simulink model "Tractive_System_model"  (R2025b)
settings: Solver=ode15s  StartTime=0  StopTime=169.89  MaxStep=1e-3  RelTol=1e-3  AbsTol=1e-6
PreLoadFcn:
  | vehicleData
undefined symbols (not defined in the file): FL, FR, RL, RR, vehicle
libraries: batteryecm_lib x281, fl_lib x86, nesl_utility x54, ee_lib x16, sdl_lib x10, SimscapeFluids_lib x3, BatteryEstimators x2, simulink x1, slpidlib x1, autolibshared x1, eePmsmFieldOrientedControl x1
(part 5 of 26)

== system Tractive_System_model/Cooling system/Subsystem1 ==
  Inverter Power_loss : Scope
      settings: ActiveDisplayYMinimum=494.41730224534911  ActiveDisplayYMaximum=494.45341613974995  DataLoggingVariableName=ScopeData3
  PS Lookup Table (2D) : fl_lib/Physical Signals/Lookup Tables/PS Lookup Table (2D)  x1=[100, 150, 200, 250, 300, 350, 400, 450, 500, 550, 600, 650, 700, 750, 800] V  x2=[100, 150, 200, 250, 300, 350, 400, 450, 500, 550, 600] A  f=|  interp_method=simscape.enum.interpolation.smooth  extrap_method=simscape.enum.extrapolation.nearest
      | [199.5, 318, 436.5, 580.5, 724.5, 899.8, 1075, 1267.5, 1460, 1692.5, 1925;
      | 230.3, 362.3, 494.3, 651.8, 809.3, 998.4, 1187.5, 1393.8, 1600, 1843.8, 2087.5;
      | 261, 406.5, 552, 723, 894, 1097, 1300, 1520, 1740, 1995, 2250;
      | 291.8, 450.8, 609.8, 794.3, 978.8, 1195.6, 1412.5, 1646.3, 1880, 2146.3, 2412.5;
      | 322.5, 495, 667.5, 865.5, 1063.5, 1294.3, 1525, 1772.5, 2020, 2297.5, 2575;
      | 353.3, 539.3, 725.3, 936.8, 1148.3, 1392.9, 1637.5, 1898.8, 2160, 2448.8, 2737.5;
      | 384, 583.5, 783, 1008, 1233, 1491.5, 1750, 2025, 2300, 2600, 2900;
      | 416.3, 629.3, 842.3, 1081.5, 1320.8, 1591.6, 1862.5, 2156.3, 2450, 2768.8, 3087.5;
      | 448.5, 675, 901.5, 1155, 1408.5, 1691.8, 1975, 2287.5, 2600, 2937.5, 3275;
      | 480.8, 720.8, 960.8, 1228.5, 1496.3, 1791.9, 2087.5, 2418.8, 2750, 3106.3, 3462.5;
      | 513, 766.5, 1020, 1302, 1584, 1892, 2200, 2550, 2900, 3275, 3650;
      | 545.3, 812.6, 1080, 1378.5, 1677, 2006, 2335, 2698.8, 3062.5, 3462.5, 3862.5;
      | 577.5, 858.8, 1140, 1455, 1770, 2120, 2470, 2847.5, 3225, 3650, 4075;
      | 609.8, 904.9, 1200, 1531.5, 1863, 2234, 2605, 2996.3, 3387.5, 3837.5, 4287.5;
      | 642, 951, 1260, 1608, 1956, 2348, 2740, 3145, 3550, 4025, 4500] W
  PS-Simulink Converter : nesl_utility/PS-Simulink Converter  PhysicalDomain=network_engine_domain  SubClassName=ps_output  LeftPortType=input  RightPortType=output  PseudoPeriodic=off  Frequencies=[]  VectorFormat=inherit  Unit=W  AffineConversion=off
  PS-Simulink Converter1 : nesl_utility/PS-Simulink Converter  PhysicalDomain=network_engine_domain  SubClassName=ps_output  LeftPortType=input  RightPortType=output  PseudoPeriodic=off  Frequencies=[]  VectorFormat=inherit  Unit=W  AffineConversion=off
  Simulink-PS Converter : nesl_utility/Simulink-PS Converter  PhysicalDomain=network_engine_domain  SubClassName=ps_input  LeftPortType=input  RightPortType=output  PseudoPeriodic=off  Frequencies=[]  NoiseDistribution=none  NoiseParameters=[]  Unit=W  AffineConversion=off  FilteringAndDerivatives=provide  SimscapeFilterOrder=1  InputFilterTimeConstant=0.001  UdotUserProvided=0
  ARMS_IN : PMIOPort  Side=Left
  VDC_IN : PMIOPort  Port=2  Side=Left
  output : PMIOPort  Port=3  Side=Right
  wires:
  PS-Simulink Converter1/1 -> Simulink-PS Converter/1
  PS-Simulink Converter/1 -> Inverter Power_loss/1
  connections:
  Simulink-PS Converter/RConn1 -- output/RConn1
  ARMS_IN/RConn1 -- PS Lookup Table (2D)/LConn2
  VDC_IN/RConn1 -- PS Lookup Table (2D)/LConn1
  PS-Simulink Converter/LConn1 -- PS Lookup Table (2D)/RConn1 -- PS-Simulink Converter1/LConn1

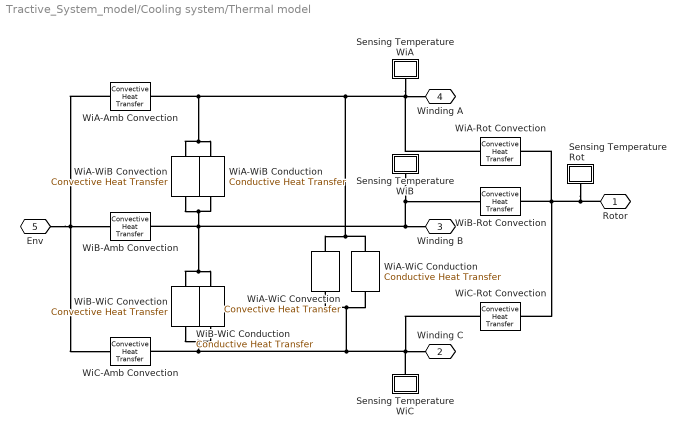
== system Tractive_System_model/Cooling system/Thermal model ==
  Sensing Temperature Rot : Subsystem
      mask Display: disp('TR')
  Sensing Temperature WiA : Subsystem
      mask Display: disp('TA')
  Sensing Temperature WiB : Subsystem
      mask Display: disp('TB')
  Sensing Temperature WiC : Subsystem
      mask Display: disp('TC')
  WiA-Amb Convection : fl_lib/Thermal/Thermal Elements/Convective Heat Transfer  thermal_type=foundation.enum.constant_variable.constant  area=0.1 m^2  heat_tr_coeff=20 W/(m^2 * K)  min_heat_tr_coeff=1e-3 W/(K*m^2)  T_specify=off  T_priority=None  T=0 K  T_nominal_specify=off  T_nominal_value=1  T_nominal_unit=K  Q_specify=off  Q_priority=None  Q=0 J/s  Q_nominal_specify=off  Q_nominal_value=1  Q_nominal_unit=J/s
  WiA-Rot Convection : fl_lib/Thermal/Thermal Elements/Convective Heat Transfer  thermal_type=foundation.enum.constant_variable.constant  area=0.02 m^2  heat_tr_coeff=200 W/(m^2 * K)  min_heat_tr_coeff=1e-3 W/(K*m^2)  T_specify=off  T_priority=None  T=0 K  T_nominal_specify=off  T_nominal_value=1  T_nominal_unit=K  Q_specify=off  Q_priority=None  Q=0 J/s  Q_nominal_specify=off  Q_nominal_value=1  Q_nominal_unit=J/s
  WiA-WiB Conduction : fl_lib/Thermal/Thermal Elements/Conductive Heat Transfer  thermal_type=foundation.enum.ConstantVariableTabulated.Constant  wall_geometry=foundation.enum.ConductionWallGeometry.Planar  area=0.002 m^2  thickness=0.1 m  d_in=0.05 m  d_out=0.1 m  L=1 m  th_cond_min=10 W/(K*m)  th_cond=80 W/(m*K)  th_cond_TLU=[413, 401, 392, 383, 371, 357, 342] W/(K*m)  temp_TLU=[200, 273, 400, 600, 800, 1000, 1200] K  T_specify=off  T_priority=None  T=0 K  T_nominal_specify=off  T_nominal_value=1  T_nominal_unit=K  Q_specify=off  Q_priority=None  Q=0 J/s  Q_nominal_specify=off  Q_nominal_value=1  Q_nominal_unit=J/s
  WiA-WiB Convection : fl_lib/Thermal/Thermal Elements/Convective Heat Transfer  thermal_type=foundation.enum.constant_variable.constant  area=0.004 m^2  heat_tr_coeff=200 W/(m^2 * K)  min_heat_tr_coeff=1e-3 W/(K*m^2)  T_specify=off  T_priority=None  T=0 K  T_nominal_specify=off  T_nominal_value=1  T_nominal_unit=K  Q_specify=off  Q_priority=None  Q=0 J/s  Q_nominal_specify=off  Q_nominal_value=1  Q_nominal_unit=J/s
  WiA-WiC Conduction : fl_lib/Thermal/Thermal Elements/Conductive Heat Transfer  thermal_type=foundation.enum.ConstantVariableTabulated.Constant  wall_geometry=foundation.enum.ConductionWallGeometry.Planar  area=0.002 m^2  thickness=0.1 m  d_in=0.05 m  d_out=0.1 m  L=1 m  th_cond_min=10 W/(K*m)  th_cond=80 W/(m*K)  th_cond_TLU=[413, 401, 392, 383, 371, 357, 342] W/(K*m)  temp_TLU=[200, 273, 400, 600, 800, 1000, 1200] K  T_specify=off  T_priority=None  T=0 K  T_nominal_specify=off  T_nominal_value=1  T_nominal_unit=K  Q_specify=off  Q_priority=None  Q=0 J/s  Q_nominal_specify=off  Q_nominal_value=1  Q_nominal_unit=J/s
  WiA-WiC Convection : fl_lib/Thermal/Thermal Elements/Convective Heat Transfer  thermal_type=foundation.enum.constant_variable.constant  area=0.004 m^2  heat_tr_coeff=200 W/(m^2 * K)  min_heat_tr_coeff=1e-3 W/(K*m^2)  T_specify=off  T_priority=None  T=0 K  T_nominal_specify=off  T_nominal_value=1  T_nominal_unit=K  Q_specify=off  Q_priority=None  Q=0 J/s  Q_nominal_specify=off  Q_nominal_value=1  Q_nominal_unit=J/s
  WiB-Amb Convection : fl_lib/Thermal/Thermal Elements/Convective Heat Transfer  thermal_type=foundation.enum.constant_variable.constant  area=0.1 m^2  heat_tr_coeff=20 W/(m^2 * K)  min_heat_tr_coeff=1e-3 W/(K*m^2)  T_specify=off  T_priority=None  T=0 K  T_nominal_specify=off  T_nominal_value=1  T_nominal_unit=K  Q_specify=off  Q_priority=None  Q=0 J/s  Q_nominal_specify=off  Q_nominal_value=1  Q_nominal_unit=J/s
  WiB-Rot Convection : fl_lib/Thermal/Thermal Elements/Convective Heat Transfer  thermal_type=foundation.enum.constant_variable.constant  area=0.02 m^2  heat_tr_coeff=200 W/(m^2 * K)  min_heat_tr_coeff=1e-3 W/(K*m^2)  T_specify=off  T_priority=None  T=0 K  T_nominal_specify=off  T_nominal_value=1  T_nominal_unit=K  Q_specify=off  Q_priority=None  Q=0 J/s  Q_nominal_specify=off  Q_nominal_value=1  Q_nominal_unit=J/s
  WiB-WiC Conduction : fl_lib/Thermal/Thermal Elements/Conductive Heat Transfer  thermal_type=foundation.enum.ConstantVariableTabulated.Constant  wall_geometry=foundation.enum.ConductionWallGeometry.Planar  area=0.002 m^2  thickness=0.1 m  d_in=0.05 m  d_out=0.1 m  L=1 m  th_cond_min=10 W/(K*m)  th_cond=80 W/(m*K)  th_cond_TLU=[413, 401, 392, 383, 371, 357, 342] W/(K*m)  temp_TLU=[200, 273, 400, 600, 800, 1000, 1200] K  T_specify=off  T_priority=None  T=0 K  T_nominal_specify=off  T_nominal_value=1  T_nominal_unit=K  Q_specify=off  Q_priority=None  Q=0 J/s  Q_nominal_specify=off  Q_nominal_value=1  Q_nominal_unit=J/s
  WiB-WiC Convection : fl_lib/Thermal/Thermal Elements/Convective Heat Transfer  thermal_type=foundation.enum.constant_variable.constant  area=0.004 m^2  heat_tr_coeff=200 W/(m^2 * K)  min_heat_tr_coeff=1e-3 W/(K*m^2)  T_specify=off  T_priority=None  T=0 K  T_nominal_specify=off  T_nominal_value=1  T_nominal_unit=K  Q_specify=off  Q_priority=None  Q=0 J/s  Q_nominal_specify=off  Q_nominal_value=1  Q_nominal_unit=J/s
  WiC-Amb Convection : fl_lib/Thermal/Thermal Elements/Convective Heat Transfer  thermal_type=foundation.enum.constant_variable.constant  area=0.1 m^2  heat_tr_coeff=20 W/(m^2 * K)  min_heat_tr_coeff=1e-3 W/(K*m^2)  T_specify=off  T_priority=None  T=0 K  T_nominal_specify=off  T_nominal_value=1  T_nominal_unit=K  Q_specify=off  Q_priority=None  Q=0 J/s  Q_nominal_specify=off  Q_nominal_value=1  Q_nominal_unit=J/s
  WiC-Rot Convection : fl_lib/Thermal/Thermal Elements/Convective Heat Transfer  thermal_type=foundation.enum.constant_variable.constant  area=0.02 m^2  heat_tr_coeff=200 W/(m^2 * K)  min_heat_tr_coeff=1e-3 W/(K*m^2)  T_specify=off  T_priority=None  T=0 K  T_nominal_specify=off  T_nominal_value=1  T_nominal_unit=K  Q_specify=off  Q_priority=None  Q=0 J/s  Q_nominal_specify=off  Q_nominal_value=1  Q_nominal_unit=J/s
  Rotor : PMIOPort  Side=Left
  Winding C : PMIOPort  Port=2  Side=Right
  Winding B : PMIOPort  Port=3  Side=Right
  Winding A : PMIOPort  Port=4  Side=Right
  Env : PMIOPort  Port=5  Side=Left
  connections:
  WiA-Rot Convection/RConn1 -- WiA-WiC Conduction/RConn1 -- WiA-WiC Convection/RConn1 -- WiA-WiB Convection/LConn1 -- WiA-WiB Conduction/LConn1 -- WiA-Amb Convection/LConn1 -- Sensing Temperature WiA/LConn1 -- Winding A/RConn1
  Rotor/RConn1 -- Sensing Temperature Rot/LConn1 -- WiC-Rot Convection/LConn1 -- WiB-Rot Convection/LConn1 -- WiA-Rot Convection/LConn1
  WiA-WiB Convection/RConn1 -- WiA-WiB Conduction/RConn1 -- Sensing Temperature WiB/LConn1 -- WiB-Rot Convection/RConn1 -- Winding B/RConn1 -- WiB-Amb Convection/LConn1 -- WiB-WiC Conduction/LConn1 -- WiB-WiC Convection/LConn1
  WiC-Rot Convection/RConn1 -- Winding C/RConn1 -- WiB-WiC Conduction/RConn1 -- WiB-WiC Convection/RConn1 -- WiC-Amb Convection/LConn1 -- WiA-WiC Convection/LConn1 -- WiA-WiC Conduction/LConn1 -- Sensing Temperature WiC/LConn1
  WiA-Amb Convection/RConn1 -- Env/RConn1 -- WiC-Amb Convection/RConn1 -- WiB-Amb Convection/RConn1

== system Tractive_System_model/Longitudinal Vehicle Dynamics1/Brakes ==
  Brake FL : sdl_lib/Brakes & Detents/Rotational/Disc Brake  r_mean=brake.padRadius mm  bore=brake.cylinderBore mm  n_pads=1  thermal_port=simscape.enum.thermaleffects.omit  mu_static=brake.sf  mu_coulomb=brake.cf  temperature_TLU=[280, 300, 320] K  mu_static_TLU=[.9, .8, .7]  mu_coulomb_TLU=[.8, .7, .6]  brkwy_vel=brake.frictionVel rad/s  visc_coef=brake.vfc N*m*s/rad  thermal_mass=50 kJ/K  temperature_specify=off  temperature_priority=High  temperature=300 K  temperature_nominal_specify=off  temperature_nominal_value=1  temperature_nominal_unit=K
  Brake FR : sdl_lib/Brakes & Detents/Rotational/Disc Brake  r_mean=brake.padRadius mm  bore=brake.cylinderBore mm  n_pads=1  thermal_port=simscape.enum.thermaleffects.omit  mu_static=brake.sf  mu_coulomb=brake.cf  temperature_TLU=[280, 300, 320] K  mu_static_TLU=[.9, .8, .7]  mu_coulomb_TLU=[.8, .7, .6]  brkwy_vel=brake.frictionVel rad/s  visc_coef=brake.vfc N*m*s/rad  thermal_mass=50 kJ/K  temperature_specify=off  temperature_priority=High  temperature=300 K  temperature_nominal_specify=off  temperature_nominal_value=1  temperature_nominal_unit=K
  Brake RL : sdl_lib/Brakes & Detents/Rotational/Disc Brake  r_mean=brake.padRadius mm  bore=brake.cylinderBore mm  n_pads=1  thermal_port=simscape.enum.thermaleffects.omit  mu_static=brake.sf  mu_coulomb=brake.cf  temperature_TLU=[280, 300, 320] K  mu_static_TLU=[.9, .8, .7]  mu_coulomb_TLU=[.8, .7, .6]  brkwy_vel=brake.frictionVel rad/s  visc_coef=brake.vfc N*m*s/rad  thermal_mass=50 kJ/K  temperature_specify=off  temperature_priority=High  temperature=300 K  temperature_nominal_specify=off  temperature_nominal_value=1  temperature_nominal_unit=K
  Brake RR : sdl_lib/Brakes & Detents/Rotational/Disc Brake  r_mean=brake.padRadius mm  bore=brake.cylinderBore mm  n_pads=1  thermal_port=simscape.enum.thermaleffects.omit  mu_static=brake.sf  mu_coulomb=brake.cf  temperature_TLU=[280, 300, 320] K  mu_static_TLU=[.9, .8, .7]  mu_coulomb_TLU=[.8, .7, .6]  brkwy_vel=brake.frictionVel rad/s  visc_coef=brake.vfc N*m*s/rad  thermal_mass=50 kJ/K  temperature_specify=off  temperature_priority=High  temperature=300 K  temperature_nominal_specify=off  temperature_nominal_value=1  temperature_nominal_unit=K
  Sensing FL : Subsystem
  Sensing FR : Subsystem
  Sensing RL : Subsystem
  Sensing RR : Subsystem
  Simscape Bus : SimscapeBus  HierarchyStrings=RR;RL;FL;FR
  BrakePrF : PMIOPort  Side=Left
  BrakePrR : PMIOPort  Port=2  Side=Left
  Shafts : PMIOPort  Port=3  Side=Right
  Out Bus Element : Outport  PortName=m  Element=FL
  Out Bus Element1 : Outport  PortName=m  Element=FR
  Out Bus Element2 : Outport  PortName=m  Element=RL
  Out Bus Element3 : Outport  PortName=m  Element=RR
  wires:
  Sensing FL/1(m) -> Out Bus Element/1
  Sensing FR/1(m) -> Out Bus Element1/1
  Sensing RL/1(m) -> Out Bus Element2/1
  Sensing RR/1(m) -> Out Bus Element3/1
  connections:
  BrakePrR/RConn1 -- Brake RL/LConn1 -- Brake RR/LConn1
  Brake FR/LConn1 -- Brake FL/LConn1 -- BrakePrF/RConn1
  Sensing FL/LConn1 -- Simscape Bus/LConn3
  Sensing FR/LConn1 -- Simscape Bus/LConn4
  Simscape Bus/LConn2 -- Sensing RL/LConn1
  Sensing RR/LConn1 -- Simscape Bus/LConn1
  Simscape Bus/RConn1 -- Shafts/RConn1
  Sensing FL/RConn1 -- Brake FL/LConn2
  Sensing FR/RConn1 -- Brake FR/LConn2
  Brake RL/LConn2 -- Sensing RL/RConn1
  Sensing RR/RConn1 -- Brake RR/LConn2

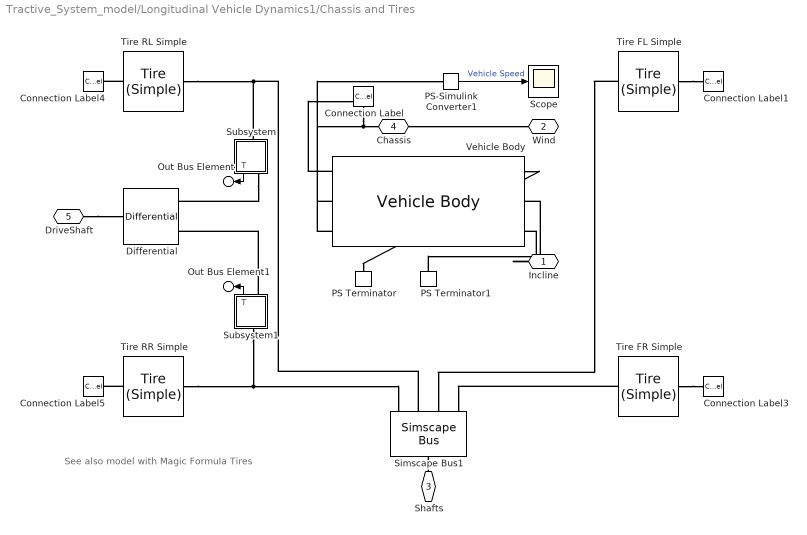
== system Tractive_System_model/Longitudinal Vehicle Dynamics1/Chassis and Tires ==
  note: See also model with Magic Formula Tires
  Connection Label{,1,3..5} (5 alike) : ConnectionLabel  Label=VehicleHub
  Differential : sdl_lib/Gears/Differential  driveshaft_location=sdl.enum.differential_orientation.right  cd_ratio=4.28  friction_model=sdl.enum.gear_friction.none  efficiency=[.85, .92]  temperature_TLU=[280, 300, 320] K  efficiency_ss_TLU=[.95, .9, .85]  efficiency_cd_TLU=[.95, .9, .85]  pwr_thr=[.001, .001] W  mu_visc=[0, 0] N*m*s/rad  model_inertia=simscape.enum.onoff.off  sun_inertia=1e-10 kg*m^2  sun_radius=0.01 m  carrier_inertia=0.001 kg*m^2  planet_inertia=0.001 kg*m^2  planet_mass=1e-10 kg  thermal_mass=50 J/K  T_init=300 K
  PS Terminator : fl_lib/Physical Signals/Sinks/PS Terminator
  PS Terminator1 : fl_lib/Physical Signals/Sinks/PS Terminator
  PS-Simulink Converter1 : nesl_utility/PS-Simulink Converter  PhysicalDomain=network_engine_domain  SubClassName=ps_output  LeftPortType=input  RightPortType=output  PseudoPeriodic=off  Frequencies=[]  VectorFormat=1-D array  Unit=1  AffineConversion=off
  Scope : Scope
      settings: ActiveDisplayYMinimum=-3.15304  ActiveDisplayYMaximum=29.55672  DataLoggingSaveFormat=Array
  Simscape Bus1 : SimscapeBus  HierarchyStrings=RR;RL;FL;FR
  Subsystem : Subsystem
  Subsystem1 : Subsystem
  Tire FL Simple : sdl_lib/Tires & Vehicles/Tire (Simple)  r_tire=vehicle.tireRollingRadius_cm cm  model_compliance=sdl.enum.compliance.off  stiffness=1e6 N/m  damping=1000 N*s/m  model_inertia=sdl.enum.model_inertia.off  tire_inertia=0.01 kg*m^2  initial_velocity=1 rad/s
      settings: InternalSimscapePortConfiguration="{\"Bottom\":[],\"Left\":[{\"id\":\"A\",\"label\":\"A\",\"type\":\"foundation.mechanical.rotational.rotational\"}],\"Right\":[{\"id\":\"H\",\"label\":\"H\",\"type\":\"foundation.mechanical.translational.translational\"}],\"Top\":[]}"
  Tire FR Simple : sdl_lib/Tires & Vehicles/Tire (Simple)  r_tire=vehicle.tireRollingRadius_cm cm  model_compliance=sdl.enum.compliance.off  stiffness=1e6 N/m  damping=1000 N*s/m  model_inertia=sdl.enum.model_inertia.off  tire_inertia=0.01 kg*m^2  initial_velocity=1 rad/s
      settings: InternalSimscapePortConfiguration="{\"Bottom\":[],\"Left\":[{\"id\":\"A\",\"label\":\"A\",\"type\":\"foundation.mechanical.rotational.rotational\"}],\"Right\":[{\"id\":\"H\",\"label\":\"H\",\"type\":\"foundation.mechanical.translational.translational\"}],\"Top\":[]}"
  Tire RL Simple : sdl_lib/Tires & Vehicles/Tire (Simple)  r_tire=vehicle.tireRollingRadius_cm cm  model_compliance=sdl.enum.compliance.off  stiffness=1e6 N/m  damping=1000 N*s/m  model_inertia=sdl.enum.model_inertia.off  tire_inertia=0.01 kg*m^2  initial_velocity=1 rad/s
      settings: InternalSimscapePortConfiguration="{\"Bottom\":[],\"Left\":[{\"id\":\"A\",\"label\":\"A\",\"type\":\"foundation.mechanical.rotational.rotational\"}],\"Right\":[{\"id\":\"H\",\"label\":\"H\",\"type\":\"foundation.mechanical.translational.translational\"}],\"Top\":[]}"
  Tire RR Simple : sdl_lib/Tires & Vehicles/Tire (Simple)  r_tire=vehicle.tireRollingRadius_cm cm  model_compliance=sdl.enum.compliance.off  stiffness=1e6 N/m  damping=1000 N*s/m  model_inertia=sdl.enum.model_inertia.off  tire_inertia=0.01 kg*m^2  initial_velocity=1 rad/s
      settings: InternalSimscapePortConfiguration="{\"Bottom\":[],\"Left\":[{\"id\":\"A\",\"label\":\"A\",\"type\":\"foundation.mechanical.rotational.rotational\"}],\"Right\":[{\"id\":\"H\",\"label\":\"H\",\"type\":\"foundation.mechanical.translational.translational\"}],\"Top\":[]}"
  Vehicle Body : sdl_lib/Tires & Vehicles/Vehicle Body  mass=vehicle.riderMass + vehicle.vehicleMass kg  n_w=2  x_f=vehicle.frontAxleDis mm  x_r=vehicle.rearAxleDis mm  y_c=vehicle.cgHeight mm  mass_var=simscape.enum.onoff.off  g=9.81 m/s^2  liftoff_warning=simscape.enum.onoff.off  area=1 m^2  Cd_var=false  Cd=0  rho=1.18 kg/m^3  model_pitch=simscape.enum.onoff.off  inertia=4000 kg*m^2  suspension_model=sdl.enum.linearTLU.linear  k_f=1e4 N/m  b_f=1e4 N*s/m  k_r=1e4 N/m  b_r=1e4 N*s/m  k_f_TLU=[-2000, -1000, 0, 1000, 2000] N  x_f_TLU=[-.4, -.2, 0, .2, .4] m  b_f_TLU=[-200, -100, 0, 100, 200] N  v_f_TLU=[-4, -2, 0, 2, 4] m/s  k_r_TLU=[-2000, -1000, 0, 1000, 2000] N  x_r_TLU=[-.4, -.2, 0, .2, .4] m  b_r_TLU=[-200, -100, 0, 100, 200] N  v_r_TLU=[-4, -2, 0, 2, 4] m/s  interp_method=simscape.enum.interpolation.linear  extrap_method=simscape.enum.extrapolation.linear  model_hardstop=simscape.enum.onoff.off  upper_bound_f=.25 m  lower_bound_f=-.25 m  stop_k_f=1e6 N/m  stop_b_f=150 N*s/m  upper_bound_r=.25 m  lower_bound_r=-.25 m  stop_k_r=1e6 N/m  stop_b_r=150 N*s/m  initial_pitch=0 rad  initial_pitch_rate=0 rad/s  v_specify=off  v_priority=High  v=12.95 m/s  v_nominal_specify=off  v_nominal_value=1  v_nominal_unit=m/s
      settings: InternalSimscapePortConfiguration="{\"Bottom\":[{\"id\":\"NR\",\"label\":\"NR\",\"type\":\"output\"},{\"id\":\"NF\",\"label\":\"NF\",\"type\":\"output\"},{\"id\":\"beta\",\"label\":\"beta\",\"type\":\"input\"}],\"Left\":[{\"id\":\"H\",\"label\":\"H\",\"type\":\"foundation.mechanical.translational.translational\"}],\"Right\":[],\"Top\":[{\"id\":\"V\",\"label\":\"V\",\"type\":\"output\"},{\"id\":\"wind\",\"label\":\"W\",\"type\":\"input\"}]}"
  Incline : PMIOPort  Side=Right
  Wind : PMIOPort  Port=2  Side=Right
  Shafts : PMIOPort  Port=3  Side=Left
  Chassis : PMIOPort  Port=4  Side=Right
  DriveShaft : PMIOPort  Port=5  Side=Left
  Out Bus Element : Outport  PortName=m  Element=tRL
  Out Bus Element1 : Outport  PortName=m  Element=tRR
  wires:
  PS-Simulink Converter1/1 -> Scope/1  "Vehicle Speed"
  Subsystem/1(T) -> Out Bus Element/1
  Subsystem1/1(T) -> Out Bus Element1/1
  connections:
  Tire RR Simple/RConn1 -- Connection Label5/LConn1
  Tire FL Simple/RConn1 -- Connection Label1/LConn1
  Tire RL Simple/RConn1 -- Connection Label4/LConn1
  Vehicle Body/LConn2 -- PS-Simulink Converter1/LConn1
  Tire FR Simple/RConn1 -- Connection Label3/LConn1
  Tire FR Simple/LConn1 -- Simscape Bus1/LConn4
  DriveShaft/RConn1 -- Differential/LConn1
  Connection Label/LConn1 -- Vehicle Body/LConn1 -- Chassis/RConn1
  Subsystem1/LConn1 -- Tire RR Simple/LConn1 -- Simscape Bus1/LConn1
  Tire FL Simple/LConn1 -- Simscape Bus1/LConn3
  Simscape Bus1/LConn2 -- Tire RL Simple/LConn1 -- Subsystem/LConn1
  Shafts/RConn1 -- Simscape Bus1/RConn1
  Incline/RConn1 -- Vehicle Body/RConn3
  Vehicle Body/LConn3 -- Wind/RConn1
  Subsystem1/RConn1 -- Differential/RConn1
  Subsystem/RConn1 -- Differential/RConn2
  Vehicle Body/RConn1 -- PS Terminator/LConn1
  PS Terminator1/LConn1 -- Vehicle Body/RConn2

== system Tractive_System_model/Longitudinal Vehicle Dynamics1/Env ==
  m : Inport
  Road Grade (rad) : Constant  Value=0
  Signal Specification : SignalSpecification  Unit=rad
  Terminator : Terminator
  Wind (m/s) : Constant  Value=0
  Bus Element Out2 : Outport  PortName=Env  Element=RoadGrade
      settings: AttributesFormatString=%<Unit>
  Bus Element Out4 : Outport  PortName=Env  Element=Wind
      settings: AttributesFormatString=%<Unit>
  wires:
  Wind (m/s)/1 -> Bus Element Out4/1
  m/1 -> Terminator/1
  Road Grade (rad)/1 -> Signal Specification/1
  Signal Specification/1 -> Bus Element Out2/1

== system Tractive_System_model/Longitudinal Vehicle Dynamics1/Sensor Subsystem ==
  AutoTerm : Terminator
  AutoTerm1 : Terminator
  Ideal Translational Motion Sensor : fl_lib/Mechanical/Mechanical Sensors/Ideal Translational Motion Sensor  reference=foundation.enum.MeasurementReference.difference  acceleration_port=false  velocity_port=true  position_port=true  offset=0 m
  Mechanical Translational Reference : fl_lib/Mechanical/Translational Elements/Mechanical Translational Reference
  PS-Simulink Converter1 : nesl_utility/PS-Simulink Converter  PhysicalDomain=network_engine_domain  SubClassName=ps_output  LeftPortType=input  RightPortType=output  PseudoPeriodic=off  Frequencies=[]  VectorFormat=1-D array  Unit=km/hr  AffineConversion=off
  PS-Simulink Converter2 : nesl_utility/PS-Simulink Converter  PhysicalDomain=network_engine_domain  SubClassName=ps_output  LeftPortType=input  RightPortType=output  PseudoPeriodic=off  Frequencies=[]  VectorFormat=1-D array  Unit=1  AffineConversion=off
  PS-Simulink Converter3 : nesl_utility/PS-Simulink Converter  PhysicalDomain=network_engine_domain  SubClassName=ps_output  LeftPortType=input  RightPortType=output  PseudoPeriodic=off  Frequencies=[]  VectorFormat=1-D array  Unit=mph  AffineConversion=off
  PS-Simulink Converter4 : nesl_utility/PS-Simulink Converter  PhysicalDomain=network_engine_domain  SubClassName=ps_output  LeftPortType=input  RightPortType=output  PseudoPeriodic=off  Frequencies=[]  VectorFormat=1-D array  Unit=m/s  AffineConversion=off
  Vehicle : PMIOPort  Side=Left
  kph : Outport  VectorParamsAs1DForOutWhenUnconnected=off
  m/s : Outport  Port=2  VectorParamsAs1DForOutWhenUnconnected=off
  wires:
  PS-Simulink Converter1/1 -> kph/1
  PS-Simulink Converter2/1 -> AutoTerm/1
  PS-Simulink Converter3/1 -> AutoTerm1/1
  PS-Simulink Converter4/1 -> m/s/1
  connections:
  Mechanical Translational Reference/LConn1 -- Ideal Translational Motion Sensor/RConn1
  PS-Simulink Converter2/LConn1 -- Ideal Translational Motion Sensor/RConn3
  Ideal Translational Motion Sensor/LConn1 -- Vehicle/RConn1
  PS-Simulink Converter3/LConn1 -- PS-Simulink Converter4/LConn1 -- Ideal Translational Motion Sensor/RConn2 -- PS-Simulink Converter1/LConn1

== system Tractive_System_model/Referenced battery pack /Accumalator ==
  Module  four : Subsystem
  Module Five1 : Subsystem
  Module One1 : Subsystem
  Module Three1 : Subsystem
  "Module Two " : Subsystem
  - : PMIOPort  Side=Left
  + : PMIOPort  Port=2  Side=Left
  connections:
  Module One1/LConn1 -- +/RConn1
  Module Five1/LConn2 -- -/RConn1
  Module  four/LConn2 -- Module Five1/LConn1
  Module One1/LConn2 -- "Module Two "/LConn1
  Module Three1/LConn2 -- Module  four/LConn1
  "Module Two "/LConn2 -- Module Three1/LConn1

== system Tractive_System_model/Referenced battery pack /SOC1 ==
  Constant2 : Constant
  Current Sensor : fl_lib/Electrical/Electrical Sensors/Current Sensor
  PS-Simulink Converter1 : nesl_utility/PS-Simulink Converter  PhysicalDomain=network_engine_domain  SubClassName=ps_output  LeftPortType=input  RightPortType=output  PseudoPeriodic=off  Frequencies=[]  VectorFormat=inherit  Unit=inherit  AffineConversion=off
  SOC : Scope
      settings: ActiveDisplayYMinimum=-1  ActiveDisplayYMaximum=1  DataLoggingVariableName=ScopeData12
  SOC Estimator (Coulomb Counting) : BatteryEstimators/SOC Estimator (Coulomb Counting)  CurrentInputPartition=on  AH=27  Ts=1  DataType=Inherit: auto
      settings: LibrarySourceBlock=|
      | batt_sl_lib/Estimators/SOC Estimator
      | (Coulomb Counting)
  Conn1 : PMIOPort  Side=Left
  Conn2 : PMIOPort  Port=2  Side=Right
  SOC batt : Outport
  wires:
  Constant2/1 -> SOC Estimator (Coulomb Counting)/2
  SOC Estimator (Coulomb Counting)/1 -> SOC/1, SOC batt/1  "Coulomb counting"
  PS-Simulink Converter1/1 -> SOC Estimator (Coulomb Counting)/1
  connections:
  Current Sensor/LConn1 -- Conn1/RConn1
  Current Sensor/RConn2 -- Conn2/RConn1
  PS-Simulink Converter1/LConn1 -- Current Sensor/RConn1

== system Tractive_System_model/Throttle controller/ Torque Reference ==
  Throtte Positon : Inport  Unit=km/hr
  Constant : Constant  Value=240
  Divide : Product  Inputs=*/
  From Workspace : FromWorkspace  Commented=on  VariableName=Current_Matrix
  Gain : Gain  Gain=0.57735026919
  Gain1 : Gain  Gain=0.83
  Product : Product
  Torque ref : Scope
      settings: ActiveDisplayYMinimum=-13.959117073448896  ActiveDisplayYMaximum=125.63205366104009  DataLoggingVariableName=ScopeData11
  percentage : Constant  Value=100
  Motortrqref : Outport  Unit=rpm  VectorParamsAs1DForOutWhenUnconnected=off
  wires:
  Throtte Positon/1 -> Divide/1
  percentage/1 -> Divide/2
  Divide/1 -> Product/2
  Constant/1 -> Product/1
  Product/1 -> Gain/1
  Gain/1 -> Gain1/1
  Gain1/1 -> Torque ref/1, Motortrqref/1

== system Tractive_System_model/Throttle controller/Control ==
  note: Is Pressure an output?
  Torque Ref : Inport
  motorspd : Inport  Port=2
  bus voltage : Inport  Port=3
  SOC : Inport  Port=4
  20Hz Lowpass Filter : TransferFcn  Denominator=[1/(2*pi*20) 1]
  Cmd Torque : Scope
      settings: ActiveDisplayYMinimum=-13.959117072781753  ActiveDisplayYMaximum=125.6320536550358
  Motor Torque : Subsystem
  MotCmdTrq : Outport
  wires:
  Motor Torque/1(motTrq) -> 20Hz Lowpass Filter/1  "MotCmdTrq"
  SOC/1 -> Motor Torque/2(SOC)
  bus voltage/1 -> Motor Torque/3(bus voltage)
  motorspd/1 -> Motor Torque/4(motorspd)
  Torque Ref/1 -> Motor Torque/1(trqReq)
  20Hz Lowpass Filter/1 -> Cmd Torque/1, MotCmdTrq/1  "Motor Speed"

== system Tractive_System_model/Controller/Control/Brake Force ==
  note: Convert requested braking torque to brake pressure
  trqReq : Inport
  Only Negative Trq : Saturate  UpperLimit=0  LowerLimit=-inf  ZeroCross=off
  trq2pressure : Gain  Gain=-3.3e6
  brkPr : Outport
  wires:
  Only Negative Trq/1 -> trq2pressure/1
  trq2pressure/1 -> brkPr/1
  trqReq/1 -> Only Negative Trq/1  "trqReq"

== system Tractive_System_model/Controller/Control/Motor Torque ==
  note: Check for Gain for regen
  note: Full torque for acceleration,
      | limited torque for deceleration (regenerative torque)
  trqReq : Inport
  1-D Lookup Table : Lookup_n-D  Commented=on  NumberOfTableDimensions=1  BreakpointsForDimension1=[0,8,15,999]  Table=[0,0,1,1]  InternalRulePriority=Speed  RndMeth=Simplest
  1-D Lookup Table1 : Lookup_n-D  Commented=on  NumberOfTableDimensions=1  BreakpointsForDimension1=[0,540,560,999]  Table=[1,1,0,0]  InternalRulePriority=Speed  RndMeth=Simplest
  1-D Lookup Table2 : Lookup_n-D  Commented=on  NumberOfTableDimensions=1  BreakpointsForDimension1=[0,0.8,0.95,1]  Table=[1,1,0,0]  InternalRulePriority=Speed  RndMeth=Simplest
  Compare To Zero : simulink/Logic and Bit Operations/Compare To Zero  relop=>  OutDataTypeStr=boolean  ZeroCross=off
  Gain accel torque : Constant
  Gain decel torque : Constant  Value=0.3
  Product : Product
  Saturation Motor Torque Limits : Saturate  UpperLimit=150  LowerLimit=-150  ZeroCross=off
  Switch : Switch  Criteria=u2 > Threshold  SaturateOnIntegerOverflow=off  InputSameDT=off
  motTrq : Outport
  wires:
  Switch/1 -> Product/1
  Gain accel torque/1 -> Switch/1
  Compare To Zero/1 -> Switch/2
  trqReq/1 -> Product/2, Compare To Zero/1
  Product/1 -> Saturation Motor Torque Limits/1
  Saturation Motor Torque Limits/1 -> motTrq/1
  Gain decel torque/1 -> Switch/3
  1-D Lookup Table/1 -> ?
  1-D Lookup Table1/1 -> ?
  1-D Lookup Table2/1 -> ?

== system Tractive_System_model/Cooling system/Cooling system /Sensing Temperature Inverter ==
  PS-Simulink Converter : nesl_utility/PS-Simulink Converter  PhysicalDomain=network_engine_domain  SubClassName=ps_output  LeftPortType=input  RightPortType=output  PseudoPeriodic=off  Frequencies=[]  VectorFormat=1-D array  Unit=degC  AffineConversion=on
  Temperature Sensor : fl_lib/Thermal/Thermal Sensors/Temperature Sensor  temperature_measure=foundation.enum.MeasurementReference.difference
  ThRef : fl_lib/Thermal/Thermal Elements/Thermal Reference
  H : PMIOPort  Side=Left
  Cooling Inverter : Outport
  wires:
  PS-Simulink Converter/1 -> Cooling Inverter/1
  connections:
  ThRef/LConn1 -- Temperature Sensor/RConn1
  H/RConn1 -- Temperature Sensor/LConn1
  Temperature Sensor/RConn2 -- PS-Simulink Converter/LConn1

== system Tractive_System_model/Cooling system/Cooling system /Subsystem ==
  "Motor Temp " : Scope
      settings: ActiveDisplayYMinimum=24.999993193295392  ActiveDisplayYMaximum=25.000005404995338  DataLoggingVariableName=ScopeData2
  PS-Simulink Converter : nesl_utility/PS-Simulink Converter  PhysicalDomain=network_engine_domain  SubClassName=ps_output  LeftPortType=input  RightPortType=output  PseudoPeriodic=off  Frequencies=[]  VectorFormat=inherit  Unit=degC  AffineConversion=on
  Temperature Sensor : fl_lib/Thermal/Thermal Sensors/Temperature Sensor  temperature_measure=foundation.enum.MeasurementReference.difference
  Thermal Reference : fl_lib/Thermal/Thermal Elements/Thermal Reference
  Conn1 : PMIOPort  Side=Left
  wires:
  PS-Simulink Converter/1 -> "Motor Temp "/1  "Motor Temperature"
  connections:
  Temperature Sensor/LConn1 -- Conn1/RConn1
  Thermal Reference/LConn1 -- Temperature Sensor/RConn1
  PS-Simulink Converter/LConn1 -- Temperature Sensor/RConn2

== system Tractive_System_model/Cooling system/Thermal model/Sensing Temperature Rot ==
  PS-Simulink Converter : nesl_utility/PS-Simulink Converter  PhysicalDomain=network_engine_domain  SubClassName=ps_output  LeftPortType=input  RightPortType=output  PseudoPeriodic=off  Frequencies=[]  VectorFormat=1-D array  Unit=degC  AffineConversion=on
  Temperature Sensor : fl_lib/Thermal/Thermal Sensors/Temperature Sensor  temperature_measure=foundation.enum.MeasurementReference.difference
  ThRef : fl_lib/Thermal/Thermal Elements/Thermal Reference
  H : PMIOPort  Side=Left
  tag scope: TR=global
  wires:
  PS-Simulink Converter/1 -> [TR]
  connections:
  Temperature Sensor/RConn2 -- PS-Simulink Converter/LConn1
  ThRef/LConn1 -- Temperature Sensor/RConn1
  H/RConn1 -- Temperature Sensor/LConn1

== system Tractive_System_model/Cooling system/Thermal model/Sensing Temperature WiA ==
  PS-Simulink Converter : nesl_utility/PS-Simulink Converter  PhysicalDomain=network_engine_domain  SubClassName=ps_output  LeftPortType=input  RightPortType=output  PseudoPeriodic=off  Frequencies=[]  VectorFormat=1-D array  Unit=degC  AffineConversion=on
  Temperature Sensor : fl_lib/Thermal/Thermal Sensors/Temperature Sensor  temperature_measure=foundation.enum.MeasurementReference.difference
  ThRef : fl_lib/Thermal/Thermal Elements/Thermal Reference
  H : PMIOPort  Side=Left
  tag scope: TA=global
  wires:
  PS-Simulink Converter/1 -> [TA]
  connections:
  H/RConn1 -- Temperature Sensor/LConn1
  ThRef/LConn1 -- Temperature Sensor/RConn1
  Temperature Sensor/RConn2 -- PS-Simulink Converter/LConn1

== system Tractive_System_model/Cooling system/Thermal model/Sensing Temperature WiB ==
  PS-Simulink Converter : nesl_utility/PS-Simulink Converter  PhysicalDomain=network_engine_domain  SubClassName=ps_output  LeftPortType=input  RightPortType=output  PseudoPeriodic=off  Frequencies=[]  VectorFormat=1-D array  Unit=degC  AffineConversion=on
  Temperature Sensor : fl_lib/Thermal/Thermal Sensors/Temperature Sensor  temperature_measure=foundation.enum.MeasurementReference.difference
  ThRef : fl_lib/Thermal/Thermal Elements/Thermal Reference
  H : PMIOPort  Side=Left
  tag scope: TB=global
  wires:
  PS-Simulink Converter/1 -> [TB]
  connections:
  ThRef/LConn1 -- Temperature Sensor/RConn1
  H/RConn1 -- Temperature Sensor/LConn1
  Temperature Sensor/RConn2 -- PS-Simulink Converter/LConn1

== system Tractive_System_model/Cooling system/Thermal model/Sensing Temperature WiC ==
  PS-Simulink Converter : nesl_utility/PS-Simulink Converter  PhysicalDomain=network_engine_domain  SubClassName=ps_output  LeftPortType=input  RightPortType=output  PseudoPeriodic=off  Frequencies=[]  VectorFormat=1-D array  Unit=degC  AffineConversion=on
  Temperature Sensor : fl_lib/Thermal/Thermal Sensors/Temperature Sensor  temperature_measure=foundation.enum.MeasurementReference.difference
  ThRef : fl_lib/Thermal/Thermal Elements/Thermal Reference
  H : PMIOPort  Side=Left
  tag scope: TC=global
  wires:
  PS-Simulink Converter/1 -> [TC]
  connections:
  H/RConn1 -- Temperature Sensor/LConn1
  ThRef/LConn1 -- Temperature Sensor/RConn1
  Temperature Sensor/RConn2 -- PS-Simulink Converter/LConn1

== system Tractive_System_model/Longitudinal Vehicle Dynamics1/Brakes/Sensing FL ==
  Mechanical Rotational Reference : fl_lib/Mechanical/Rotational Elements/Mechanical Rotational Reference
  Motion Sensor : fl_lib/Mechanical/Mechanical Sensors/Ideal Rotational Motion Sensor  reference=foundation.enum.MeasurementReference.difference  acceleration_port=false  velocity_port=true  position_port=true  wrap_angle=simscape.enum.onoff.off  offset=0 rad
  PS Terminator : fl_lib/Physical Signals/Sinks/PS Terminator
  PS-Simulink Converter : nesl_utility/PS-Simulink Converter  PhysicalDomain=network_engine_domain  SubClassName=ps_output  LeftPortType=input  RightPortType=output  PseudoPeriodic=off  Frequencies=[]  VectorFormat=inherit  Unit=inherit  AffineConversion=off
  PS-Simulink Converter1 : nesl_utility/PS-Simulink Converter  PhysicalDomain=network_engine_domain  SubClassName=ps_output  LeftPortType=input  RightPortType=output  PseudoPeriodic=off  Frequencies=[]  VectorFormat=inherit  Unit=inherit  AffineConversion=off
  Torque Sensor : fl_lib/Mechanical/Mechanical Sensors/Ideal Torque Sensor
  C : PMIOPort  Side=Left
  R : PMIOPort  Port=2  Side=Right
  Out Bus Element : Outport  PortName=m  Element=brkTrqFL
  Out Bus Element1 : Outport  PortName=m  Element=wFL
  wires:
  PS-Simulink Converter1/1 -> Out Bus Element1/1  "w"
  PS-Simulink Converter/1 -> Out Bus Element/1  "trq"
  connections:
  Motion Sensor/RConn3 -- PS Terminator/LConn1
  PS-Simulink Converter1/LConn1 -- Motion Sensor/RConn2
  Motion Sensor/RConn1 -- Mechanical Rotational Reference/LConn1
  Torque Sensor/RConn1 -- C/RConn1
  Motion Sensor/LConn1 -- Torque Sensor/LConn1 -- R/RConn1
  PS-Simulink Converter/LConn1 -- Torque Sensor/RConn2

== system Tractive_System_model/Longitudinal Vehicle Dynamics1/Brakes/Sensing FR ==
  Mechanical Rotational Reference : fl_lib/Mechanical/Rotational Elements/Mechanical Rotational Reference
  Motion Sensor : fl_lib/Mechanical/Mechanical Sensors/Ideal Rotational Motion Sensor  reference=foundation.enum.MeasurementReference.difference  acceleration_port=false  velocity_port=true  position_port=true  wrap_angle=simscape.enum.onoff.off  offset=0 rad
  PS Terminator : fl_lib/Physical Signals/Sinks/PS Terminator
  PS-Simulink Converter : nesl_utility/PS-Simulink Converter  PhysicalDomain=network_engine_domain  SubClassName=ps_output  LeftPortType=input  RightPortType=output  PseudoPeriodic=off  Frequencies=[]  VectorFormat=inherit  Unit=inherit  AffineConversion=off
  PS-Simulink Converter1 : nesl_utility/PS-Simulink Converter  PhysicalDomain=network_engine_domain  SubClassName=ps_output  LeftPortType=input  RightPortType=output  PseudoPeriodic=off  Frequencies=[]  VectorFormat=inherit  Unit=inherit  AffineConversion=off
  Torque Sensor : fl_lib/Mechanical/Mechanical Sensors/Ideal Torque Sensor
  C : PMIOPort  Side=Left
  R : PMIOPort  Port=2  Side=Right
  Out Bus Element : Outport  PortName=m  Element=brkTrqFR
  Out Bus Element1 : Outport  PortName=m  Element=wFR
  wires:
  PS-Simulink Converter/1 -> Out Bus Element/1  "trq"
  PS-Simulink Converter1/1 -> Out Bus Element1/1  "w"
  connections:
  PS-Simulink Converter/LConn1 -- Torque Sensor/RConn2
  R/RConn1 -- Torque Sensor/LConn1 -- Motion Sensor/LConn1
  Torque Sensor/RConn1 -- C/RConn1
  Motion Sensor/RConn1 -- Mechanical Rotational Reference/LConn1
  PS-Simulink Converter1/LConn1 -- Motion Sensor/RConn2
  Motion Sensor/RConn3 -- PS Terminator/LConn1

== system Tractive_System_model/Longitudinal Vehicle Dynamics1/Brakes/Sensing RL ==
  Mechanical Rotational Reference : fl_lib/Mechanical/Rotational Elements/Mechanical Rotational Reference
  Motion Sensor : fl_lib/Mechanical/Mechanical Sensors/Ideal Rotational Motion Sensor  reference=foundation.enum.MeasurementReference.difference  acceleration_port=false  velocity_port=true  position_port=true  wrap_angle=simscape.enum.onoff.off  offset=0 rad
  PS Terminator : fl_lib/Physical Signals/Sinks/PS Terminator
  PS-Simulink Converter : nesl_utility/PS-Simulink Converter  PhysicalDomain=network_engine_domain  SubClassName=ps_output  LeftPortType=input  RightPortType=output  PseudoPeriodic=off  Frequencies=[]  VectorFormat=inherit  Unit=inherit  AffineConversion=off
  PS-Simulink Converter1 : nesl_utility/PS-Simulink Converter  PhysicalDomain=network_engine_domain  SubClassName=ps_output  LeftPortType=input  RightPortType=output  PseudoPeriodic=off  Frequencies=[]  VectorFormat=inherit  Unit=inherit  AffineConversion=off
  Torque Sensor : fl_lib/Mechanical/Mechanical Sensors/Ideal Torque Sensor
  C : PMIOPort  Side=Left
  R : PMIOPort  Port=2  Side=Right
  Out Bus Element : Outport  PortName=m  Element=brkTrqRL
  Out Bus Element1 : Outport  PortName=m  Element=wRL
  wires:
  PS-Simulink Converter/1 -> Out Bus Element/1  "trq"
  PS-Simulink Converter1/1 -> Out Bus Element1/1  "w"
  connections:
  PS-Simulink Converter/LConn1 -- Torque Sensor/RConn2
  Torque Sensor/LConn1 -- Motion Sensor/LConn1 -- R/RConn1
  Torque Sensor/RConn1 -- C/RConn1
  Motion Sensor/RConn1 -- Mechanical Rotational Reference/LConn1
  PS-Simulink Converter1/LConn1 -- Motion Sensor/RConn2
  Motion Sensor/RConn3 -- PS Terminator/LConn1

== system Tractive_System_model/Longitudinal Vehicle Dynamics1/Brakes/Sensing RR ==
  Mechanical Rotational Reference : fl_lib/Mechanical/Rotational Elements/Mechanical Rotational Reference
  Motion Sensor : fl_lib/Mechanical/Mechanical Sensors/Ideal Rotational Motion Sensor  reference=foundation.enum.MeasurementReference.difference  acceleration_port=false  velocity_port=true  position_port=true  wrap_angle=simscape.enum.onoff.off  offset=0 rad
  PS Terminator : fl_lib/Physical Signals/Sinks/PS Terminator
  PS-Simulink Converter : nesl_utility/PS-Simulink Converter  PhysicalDomain=network_engine_domain  SubClassName=ps_output  LeftPortType=input  RightPortType=output  PseudoPeriodic=off  Frequencies=[]  VectorFormat=inherit  Unit=inherit  AffineConversion=off
  PS-Simulink Converter1 : nesl_utility/PS-Simulink Converter  PhysicalDomain=network_engine_domain  SubClassName=ps_output  LeftPortType=input  RightPortType=output  PseudoPeriodic=off  Frequencies=[]  VectorFormat=inherit  Unit=inherit  AffineConversion=off
  Torque Sensor : fl_lib/Mechanical/Mechanical Sensors/Ideal Torque Sensor
  C : PMIOPort  Side=Left
  R : PMIOPort  Port=2  Side=Right
  Out Bus Element : Outport  PortName=m  Element=brqTrqRR
  Out Bus Element1 : Outport  PortName=m  Element=wRR
  wires:
  PS-Simulink Converter1/1 -> Out Bus Element1/1  "w"
  PS-Simulink Converter/1 -> Out Bus Element/1  "trq"
  connections:
  Motion Sensor/RConn3 -- PS Terminator/LConn1
  PS-Simulink Converter1/LConn1 -- Motion Sensor/RConn2
  Motion Sensor/RConn1 -- Mechanical Rotational Reference/LConn1
  Torque Sensor/RConn1 -- C/RConn1
  Motion Sensor/LConn1 -- Torque Sensor/LConn1 -- R/RConn1
  PS-Simulink Converter/LConn1 -- Torque Sensor/RConn2

== system Tractive_System_model/Longitudinal Vehicle Dynamics1/Chassis and Tires/Subsystem ==
  PS-Simulink Converter : nesl_utility/PS-Simulink Converter  PhysicalDomain=network_engine_domain  SubClassName=ps_output  LeftPortType=input  RightPortType=output  PseudoPeriodic=off  Frequencies=[]  VectorFormat=inherit  Unit=inherit  AffineConversion=off
  Torque Sensor Motor RL : fl_lib/Mechanical/Mechanical Sensors/Ideal Torque Sensor
  C : PMIOPort  Side=Left
  R : PMIOPort  Port=2  Side=Right
  T : Outport
  wires:
  PS-Simulink Converter/1 -> T/1
  connections:
  Torque Sensor Motor RL/RConn1 -- C/RConn1
  Torque Sensor Motor RL/LConn1 -- R/RConn1
  PS-Simulink Converter/LConn1 -- Torque Sensor Motor RL/RConn2

== system Tractive_System_model/Longitudinal Vehicle Dynamics1/Chassis and Tires/Subsystem1 ==
  PS-Simulink Converter : nesl_utility/PS-Simulink Converter  PhysicalDomain=network_engine_domain  SubClassName=ps_output  LeftPortType=input  RightPortType=output  PseudoPeriodic=off  Frequencies=[]  VectorFormat=inherit  Unit=inherit  AffineConversion=off
  Torque Sensor Motor RL : fl_lib/Mechanical/Mechanical Sensors/Ideal Torque Sensor
  C : PMIOPort  Side=Left
  R : PMIOPort  Port=2  Side=Right
  T : Outport
  wires:
  PS-Simulink Converter/1 -> T/1
  connections:
  PS-Simulink Converter/LConn1 -- Torque Sensor Motor RL/RConn2
  Torque Sensor Motor RL/LConn1 -- R/RConn1
  Torque Sensor Motor RL/RConn1 -- C/RConn1
